simulink model "EnergyMonitoringSystem"  (R2024a)
settings: Solver=VariableStepAuto  StartTime=0.0  StopTime=10.0  RelTol=1e-3
settings Model: Creator=dogba  LastModifiedBy=dogba

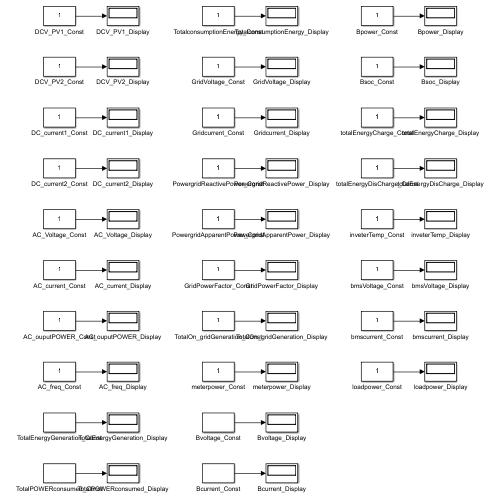
[thumbnail: Simulink's stored preview of the top-level diagram]
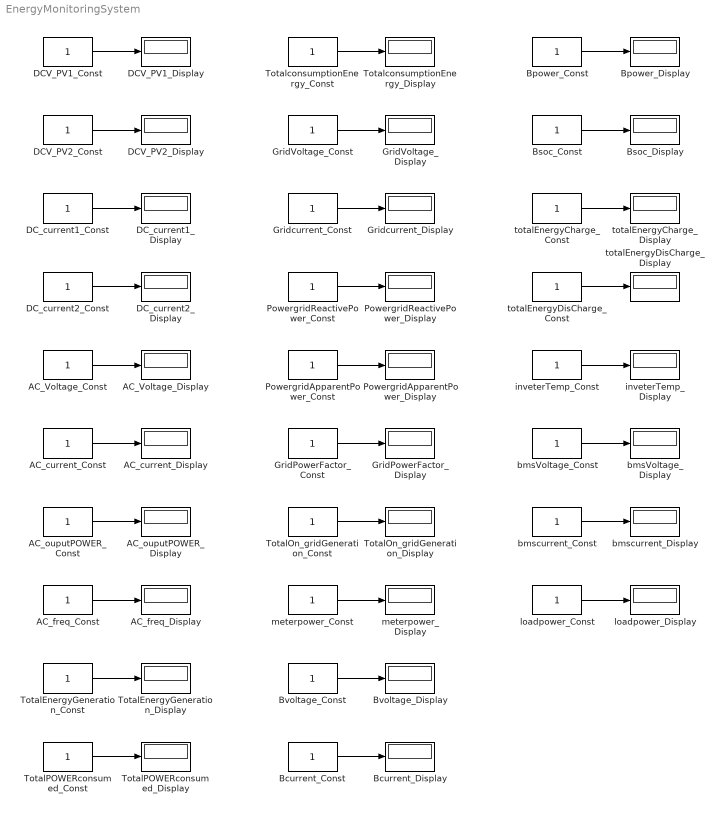
== system EnergyMonitoringSystem ==
  AC_Voltage_Const : Constant
  AC_Voltage_Display : Display
  AC_current_Const : Constant
  AC_current_Display : Display
  AC_freq_Const : Constant
  AC_freq_Display : Display
  AC_ouputPOWER_Const : Constant
  AC_ouputPOWER_Display : Display
  Bcurrent_Const : Constant
  Bcurrent_Display : Display
  Bpower_Const : Constant
  Bpower_Display : Display
  Bsoc_Const : Constant
  Bsoc_Display : Display
  Bvoltage_Const : Constant
  Bvoltage_Display : Display
  DCV_PV1_Const : Constant
  DCV_PV1_Display : Display
  DCV_PV2_Const : Constant
  DCV_PV2_Display : Display
  DC_current1_Const : Constant
  DC_current1_Display : Display
  DC_current2_Const : Constant
  DC_current2_Display : Display
  GridPowerFactor_Const : Constant
  GridPowerFactor_Display : Display
  GridVoltage_Const : Constant
  GridVoltage_Display : Display
  Gridcurrent_Const : Constant
  Gridcurrent_Display : Display
  PowergridApparentPower_Const : Constant
  PowergridApparentPower_Display : Display
  PowergridReactivePower_Const : Constant
  PowergridReactivePower_Display : Display
  TotalEnergyGeneration_Const : Constant
  TotalEnergyGeneration_Display : Display
  TotalOn_gridGeneration_Const : Constant
  TotalOn_gridGeneration_Display : Display
  TotalPOWERconsumed_Const : Constant
  TotalPOWERconsumed_Display : Display
  TotalconsumptionEnergy_Const : Constant
  TotalconsumptionEnergy_Display : Display
  bmsVoltage_Const : Constant
  bmsVoltage_Display : Display
  bmscurrent_Const : Constant
  bmscurrent_Display : Display
  inveterTemp_Const : Constant
  inveterTemp_Display : Display
  loadpower_Const : Constant
  loadpower_Display : Display
  meterpower_Const : Constant
  meterpower_Display : Display
  totalEnergyCharge_Const : Constant
  totalEnergyCharge_Display : Display
  totalEnergyDisCharge_Const : Constant
  totalEnergyDisCharge_Display : Display
  wires:
  DCV_PV1_Const/1 -> DCV_PV1_Display/1
  DCV_PV2_Const/1 -> DCV_PV2_Display/1
  DC_current1_Const/1 -> DC_current1_Display/1
  DC_current2_Const/1 -> DC_current2_Display/1
  AC_Voltage_Const/1 -> AC_Voltage_Display/1
  AC_current_Const/1 -> AC_current_Display/1
  AC_ouputPOWER_Const/1 -> AC_ouputPOWER_Display/1
  AC_freq_Const/1 -> AC_freq_Display/1
  TotalEnergyGeneration_Const/1 -> TotalEnergyGeneration_Display/1
  TotalPOWERconsumed_Const/1 -> TotalPOWERconsumed_Display/1
  TotalconsumptionEnergy_Const/1 -> TotalconsumptionEnergy_Display/1
  GridVoltage_Const/1 -> GridVoltage_Display/1
  Gridcurrent_Const/1 -> Gridcurrent_Display/1
  PowergridReactivePower_Const/1 -> PowergridReactivePower_Display/1
  PowergridApparentPower_Const/1 -> PowergridApparentPower_Display/1
  GridPowerFactor_Const/1 -> GridPowerFactor_Display/1
  TotalOn_gridGeneration_Const/1 -> TotalOn_gridGeneration_Display/1
  meterpower_Const/1 -> meterpower_Display/1
  Bvoltage_Const/1 -> Bvoltage_Display/1
  Bcurrent_Const/1 -> Bcurrent_Display/1
  Bpower_Const/1 -> Bpower_Display/1
  Bsoc_Const/1 -> Bsoc_Display/1
  totalEnergyCharge_Const/1 -> totalEnergyCharge_Display/1
  totalEnergyDisCharge_Const/1 -> totalEnergyDisCharge_Display/1
  inveterTemp_Const/1 -> inveterTemp_Display/1
  bmsVoltage_Const/1 -> bmsVoltage_Display/1
  bmscurrent_Const/1 -> bmscurrent_Display/1
  loadpower_Const/1 -> loadpower_Display/1
